simulink library "CTRL_UP"  (R2023b)
settings: Solver=VariableStepAuto  StartTime=0.0  StopTime=10.0  RelTol=1e-3
libraries: CTRL_UP_SLISUR x1, CTRL_UP_YAWACC x1, CTRL_UP_YTDES x1, VUT_lib x1
settings Model: Creator=blatak  LastModifiedBy=blatak

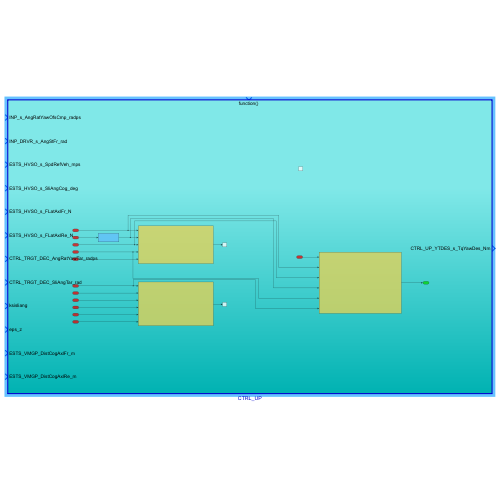
[thumbnail: Simulink's stored preview of the top-level diagram]
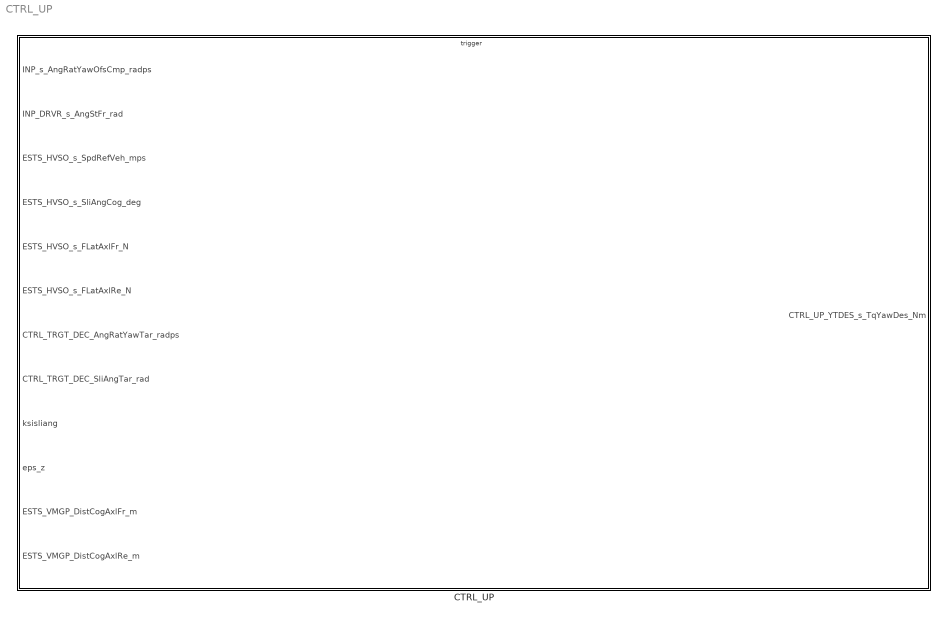
== system CTRL_UP ==
  CTRL_UP : Subsystem  TreatAsAtomicUnit=on

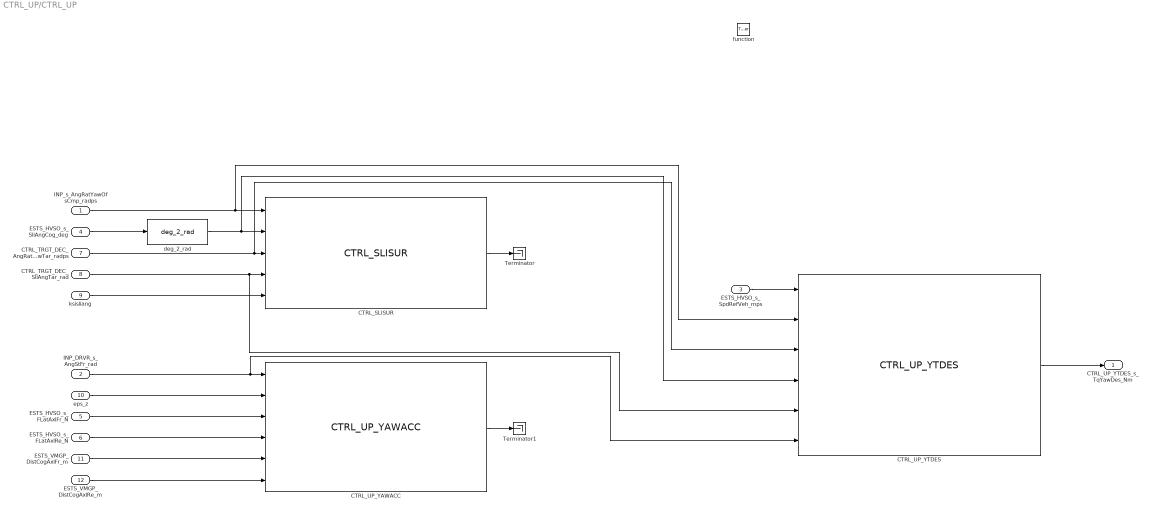
== system CTRL_UP/CTRL_UP ==
  INP_s_AngRatYawOfsCmp_radps : Inport
  INP_DRVR_s_AngStFr_rad : Inport  Port=2
  ESTS_HVSO_s_SpdRefVeh_mps : Inport  Port=3
  ESTS_HVSO_s_SliAngCog_deg : Inport  Port=4
  ESTS_HVSO_s_FLatAxlFr_N : Inport  Port=5
  ESTS_HVSO_s_FLatAxlRe_N : Inport  Port=6
  CTRL_TRGT_DEC_AngRatYawTar_radps : Inport  Port=7
  CTRL_TRGT_DEC_SliAngTar_rad : Inport  Port=8
  ksisliang : Inport  Port=9
  eps_z : Inport  Port=10
  ESTS_VMGP_DistCogAxlFr_m : Inport  Port=11
  ESTS_VMGP_DistCogAxlRe_m : Inport  Port=12
  function : TriggerPort  TriggerType=function-call  VariantControl=(inherit)
  CTRL_SLISUR : CTRL_UP_SLISUR/CTRL_SLISUR  SystemSampleTime=-1  VariantActivationTime=update diagram  AllowFlexibleInterface=on  Latency=0  AutoFrameSizeCalculation=off
  CTRL_UP_YAWACC : CTRL_UP_YAWACC/CTRL_UP_YAWACC  SystemSampleTime=-1  VariantActivationTime=update diagram  AllowFlexibleInterface=on  Latency=0  AutoFrameSizeCalculation=off
  CTRL_UP_YTDES : CTRL_UP_YTDES/CTRL_UP_YTDES  SystemSampleTime=-1  VariantActivationTime=update diagram  AllowFlexibleInterface=on  Latency=0  AutoFrameSizeCalculation=off
  Terminator : Terminator
  Terminator1 : Terminator
  deg_2_rad : VUT_lib/deg_2_rad  SystemSampleTime=-1  VariantActivationTime=update diagram  AllowFlexibleInterface=on  Latency=0  AutoFrameSizeCalculation=off
  CTRL_UP_YTDES_s_TqYawDes_Nm : Outport
  wires:
  INP_s_AngRatYawOfsCmp_radps/1 -> CTRL_SLISUR/1, CTRL_UP_YTDES/2
  CTRL_TRGT_DEC_AngRatYawTar_radps/1 -> CTRL_UP_YTDES/3, CTRL_SLISUR/3
  CTRL_TRGT_DEC_SliAngTar_rad/1 -> CTRL_SLISUR/4, CTRL_UP_YTDES/5
  ksisliang/1 -> CTRL_SLISUR/5
  INP_DRVR_s_AngStFr_rad/1 -> CTRL_UP_YTDES/6, CTRL_UP_YAWACC/1
  eps_z/1 -> CTRL_UP_YAWACC/2
  ESTS_HVSO_s_FLatAxlFr_N/1 -> CTRL_UP_YAWACC/3
  ESTS_HVSO_s_FLatAxlRe_N/1 -> CTRL_UP_YAWACC/4
  ESTS_VMGP_DistCogAxlFr_m/1 -> CTRL_UP_YAWACC/5
  ESTS_VMGP_DistCogAxlRe_m/1 -> CTRL_UP_YAWACC/6
  ESTS_HVSO_s_SpdRefVeh_mps/1 -> CTRL_UP_YTDES/1
  CTRL_SLISUR/1 -> Terminator/1
  CTRL_UP_YAWACC/1 -> Terminator1/1
  CTRL_UP_YTDES/1 -> CTRL_UP_YTDES_s_TqYawDes_Nm/1
  ESTS_HVSO_s_SliAngCog_deg/1 -> deg_2_rad/1
  deg_2_rad/1 -> CTRL_UP_YTDES/4, CTRL_SLISUR/2
